simulink library "MIDG_labels_lib"  (Simulink 6.6)
libraries: simulink x1
settings Model: Creator=cbuttril  LastModifiedBy=cbuttril

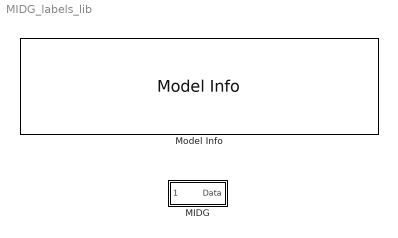
== system MIDG_labels_lib ==
  MIDG : Subsystem
  Model Info : simulink/Model-Wide Utilities/Model Info  SystemSampleTime=-1  InitialBlockCM=None  BlockCM=None  Frame=on  DisplayStringWithTags=|  HorizontalTextAlignment=Center  LeftAlignmentValue=0.5  SourceBlockDiagram=MIDG_lib  TagMaxNumber=20
      | Developed using Matlab Release 2007a
      | 
      | SVN:%<ModelVersion>
      | Last modifed by %<LastModifiedBy> on %<LastModificationDate>

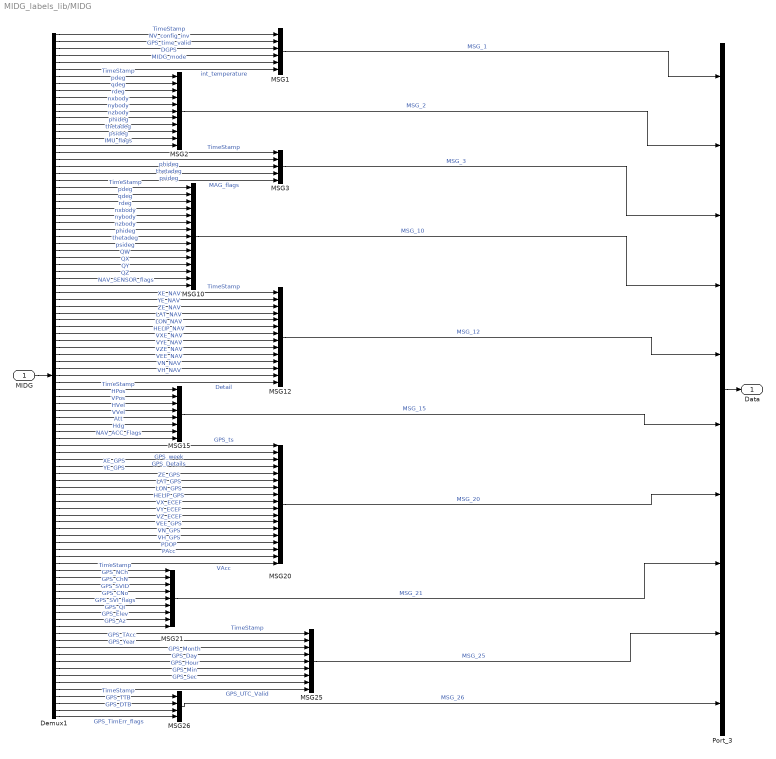
== system MIDG_labels_lib/MIDG ==
  MIDG : Inport  PortDimensions=99
  Demux1 : Demux  Outputs=99
  MSG1 : BusCreator  Inputs=6
  MSG10 : BusCreator  Inputs=15
  MSG12 : BusCreator  Inputs=14
  MSG15 : BusCreator  Inputs=8
  MSG2 : BusCreator  Inputs=11
  MSG20 : BusCreator  Inputs=18
  MSG21 : BusCreator  Inputs=9
  MSG25 : BusCreator  Inputs=9
  MSG26 : BusCreator
  MSG3 : BusCreator  Inputs=5
  Port_3 : BusCreator  Inputs=10
  Data : Outport  PortDimensions=99
  wires:
  Port_3/1 -> Data/1
  Demux1/96 -> MSG26/1  "TimeStamp"
  Demux1/97 -> MSG26/2  "GPS_TTB"
  Demux1/98 -> MSG26/3  "GPS_DTB"
  Demux1/99 -> MSG26/4  "GPS_TimErr_flags"
  Demux1/94 -> MSG25/8  "GPS_Sec"
  Demux1/95 -> MSG25/9  "GPS_UTC_Valid"
  Demux1/93 -> MSG25/7  "GPS_Min"
  Demux1/92 -> MSG25/6  "GPS_Hour"
  Demux1/91 -> MSG25/5  "GPS_Day"
  Demux1/90 -> MSG25/4  "GPS_Month"
  Demux1/89 -> MSG25/3  "GPS_Year"
  Demux1/88 -> MSG25/2  "GPS_TAcc"
  Demux1/87 -> MSG25/1  "TimeStamp"
  Demux1/78 -> MSG21/1  "TimeStamp"
  Demux1/85 -> MSG21/8  "GPS_Elev"
  Demux1/79 -> MSG21/2  "GPS_NCh"
  Demux1/80 -> MSG21/3  "GPS_ChN"
  Demux1/81 -> MSG21/4  "GPS_SVID"
  Demux1/82 -> MSG21/5  "GPS_CNo"
  Demux1/83 -> MSG21/6  "GPS_SVI_flags"
  Demux1/84 -> MSG21/7  "GPS_QI"
  Demux1/86 -> MSG21/9  "GPS_Az"
  Demux1/60 -> MSG20/1  "GPS_ts"
  Demux1/61 -> MSG20/2  "GPS_week"
  Demux1/62 -> MSG20/3  "GPS_Details"
  Demux1/77 -> MSG20/18  "VAcc"
  Demux1/76 -> MSG20/17  "PAcc"
  Demux1/75 -> MSG20/16  "PDOP"
  Demux1/74 -> MSG20/15  "VH_GPS"
  Demux1/73 -> MSG20/14  "VN_GPS"
  Demux1/72 -> MSG20/13  "VEE_GPS"
  Demux1/71 -> MSG20/12  "VZ_ECEF"
  Demux1/70 -> MSG20/11  "VY_ECEF"
  Demux1/69 -> MSG20/10  "VX_ECEF"
  Demux1/68 -> MSG20/9  "HELIP_GPS"
  Demux1/67 -> MSG20/8  "LON_GPS"
  Demux1/66 -> MSG20/7  "LAT_GPS"
  Demux1/65 -> MSG20/6  "ZE_GPS"
  Demux1/64 -> MSG20/5  "YE_GPS"
  Demux1/63 -> MSG20/4  "XE_GPS"
  Demux1/52 -> MSG15/1  "TimeStamp"
  Demux1/59 -> MSG15/8  "NAV_ACC_Flags"
  Demux1/53 -> MSG15/2  "HPos"
  Demux1/54 -> MSG15/3  "VPos"
  Demux1/55 -> MSG15/4  "HVel"
  Demux1/56 -> MSG15/5  "VVel"
  Demux1/57 -> MSG15/6  "Att"
  Demux1/58 -> MSG15/7  "Hdg"
  Demux1/41 -> MSG12/4  "ZE_NAV"
  Demux1/42 -> MSG12/5  "LAT_NAV"
  Demux1/43 -> MSG12/6  "LON_NAV"
  Demux1/44 -> MSG12/7  "HELIP_NAV"
  Demux1/45 -> MSG12/8  "VXE_NAV"
  Demux1/46 -> MSG12/9  "VYE_NAV"
  Demux1/47 -> MSG12/10  "VZE_NAV"
  Demux1/48 -> MSG12/11  "VEE_NAV"
  Demux1/49 -> MSG12/12  "VN_NAV"
  Demux1/50 -> MSG12/13  "VH_NAV"
  Demux1/51 -> MSG12/14  "Detail"
  Demux1/40 -> MSG12/3  "YE_NAV"
  Demux1/39 -> MSG12/2  "XE_NAV"
  Demux1/38 -> MSG12/1  "TimeStamp"
  Demux1/37 -> MSG10/15  "NAV_SENSOR_flags"
  Demux1/36 -> MSG10/14  "QZ"
  Demux1/35 -> MSG10/13  "QY"
  Demux1/34 -> MSG10/12  "QX"
  Demux1/33 -> MSG10/11  "QW"
  Demux1/22 -> MSG3/5  "MAG_flags"
  Demux1/17 -> MSG2/11  "IMU_flags"
  Demux1/1 -> MSG1/1  "TimeStamp"
  Demux1/2 -> MSG1/2  "NV_config_inv"
  Demux1/3 -> MSG1/3  "GPS_time_valid"
  Demux1/4 -> MSG1/4  "DGPS"
  Demux1/5 -> MSG1/5  "MIDG_mode"
  Demux1/6 -> MSG1/6  "int_temperature"
  MSG21/1 -> Port_3/8  "MSG_21"
  MSG20/1 -> Port_3/7  "MSG_20"
  MSG10/1 -> Port_3/4  "MSG_10"
  MSG26/1 -> Port_3/10  "MSG_26"
  MSG25/1 -> Port_3/9  "MSG_25"
  MSG15/1 -> Port_3/6  "MSG_15"
  MSG12/1 -> Port_3/5  "MSG_12"
  MSG3/1 -> Port_3/3  "MSG_3"
  MSG2/1 -> Port_3/2  "MSG_2"
  MSG1/1 -> Port_3/1  "MSG_1"
  Demux1/7 -> MSG2/1  "TimeStamp"
  Demux1/8 -> MSG2/2  "pdeg"
  Demux1/9 -> MSG2/3  "qdeg"
  Demux1/10 -> MSG2/4  "rdeg"
  Demux1/11 -> MSG2/5  "nxbody"
  Demux1/12 -> MSG2/6  "nybody"
  Demux1/13 -> MSG2/7  "nzbody"
  Demux1/14 -> MSG2/8  "phideg"
  Demux1/15 -> MSG2/9  "thetadeg"
  Demux1/16 -> MSG2/10  "psideg"
  Demux1/18 -> MSG3/1  "TimeStamp"
  Demux1/19 -> MSG3/2  "phideg"
  Demux1/20 -> MSG3/3  "thetadeg"
  Demux1/21 -> MSG3/4  "psideg"
  Demux1/23 -> MSG10/1  "TimeStamp"
  Demux1/24 -> MSG10/2  "pdeg"
  Demux1/25 -> MSG10/3  "qdeg"
  Demux1/26 -> MSG10/4  "rdeg"
  Demux1/27 -> MSG10/5  "nxbody"
  Demux1/28 -> MSG10/6  "nybody"
  Demux1/29 -> MSG10/7  "nzbody"
  Demux1/30 -> MSG10/8  "phideg"
  Demux1/31 -> MSG10/9  "thetadeg"
  Demux1/32 -> MSG10/10  "psideg"
  MIDG/1 -> Demux1/1
